simulink model "WAMVmodel_2017b"  (R2017b)
settings: Solver=ode23  StartTime=0.0  StopTime=param.tf  MaxStep=0.1  RelTol=1e-4  EnableMultiTasking=on
undefined symbols (not defined in the file or in its folder): param
settings Model: Creator=tristan  LastModifiedBy=masom
settings DataIOCC: LimitDataPoints=on  SaveFormat=Array  SignalLoggingSaveFormat=ModelDataLogs
settings OptimizationCC: ExpressionDepthLimit=2147483647  LifeSpan=inf
settings DebuggingCC: UnderspecifiedInitializationDetection=Classic  MergeDetectMultiDrivingBlocksExec=none  SolverPrmCheckMsg=warning  FcnCallInpInsideContextMsg=warning  StateNameClashWarn=warning  SFUnexpectedBacktrackingDiag=warning  SFNoUnconditionalDefaultTransitionDiag=warning  SFExecutionAtInitializationDiag=none
settings HardwareCC: ProdBitPerPointer=32  ProdBitPerSizeT=32  ProdBitPerPtrDiffT=32  ProdLargestAtomicFloat=None  ProdIntDivRoundTo=Undefined  ProdEndianess=Unspecified  ProdWordSize=32  ProdHWDeviceType=32-bit Generic
settings ModelReferenceCC: PropagateSignalLabelsOutOfModel=off
settings CodeAppCC: StateflowObjectComments=on
settings GRTTargetCC: TargetLangStandard=C89/C90 (ANSI)  GeneratePreprocessorConditionals=Disable all  CombineOutputUpdateFcns=off  GRTInterface=on
settings ConfigComp: CovMetricSettings=dw  CovHtmlReporting=on  CovSaveCumulativeToWorkspaceVar=on  CovSaveSingleToWorkspaceVar=on  CovExternalEMLEnable=off

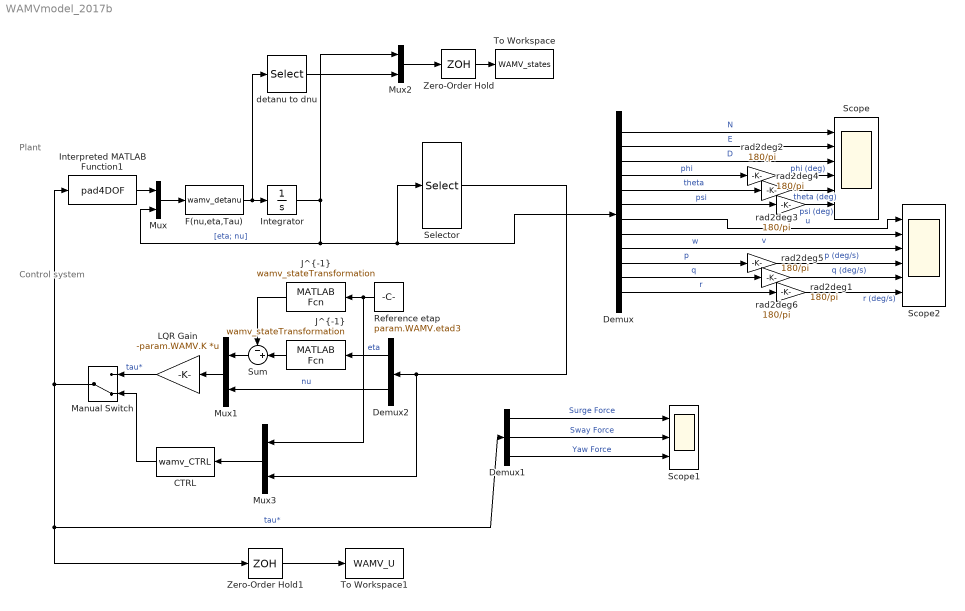
== system WAMVmodel_2017b ==
  note: Control system
  note: Plant
  CTRL : MATLABFcn  MATLABFcn=wamv_CTRL  OutputDimensions=3
  Demux : Demux  Outputs=12
  Demux1 : Demux  Outputs=3
  Demux2 : Demux  Outputs=[3,3]
  F(nu,eta,Tau) : MATLABFcn  MATLABFcn=wamv_detanu  OutputDimensions=12
  Integrator : Integrator  InitialCondition=param.WAMV.etai
  Interpreted MATLAB Function1 : MATLABFcn  MATLABFcn=pad4DOF  OutputDimensions=6
  "J^{-1}" : MATLABFcn  MATLABFcn=wamv_stateTransformation  OutputDimensions=3
  "J^{-1} " : MATLABFcn  MATLABFcn=wamv_stateTransformation  OutputDimensions=3
  LQR Gain : Gain  Gain=-param.WAMV.K  Multiplication=Matrix(K*u)
  Manual Switch : ManualSwitch  CurrentSetting=0
  Mux{,1..3} (4 alike) : Mux  Inputs=2
  Reference etap : Constant  Value=param.WAMV.etad3
  Scope : Scope  NumInputPorts=6
  Scope1 : Scope  NumInputPorts=3
  Scope2 : Scope  NumInputPorts=6
  Selector : Selector  InputPortWidth=12  IndexOptions=Index vector (dialog)  Indices=[1 2 6 7 8 12]  OutputSizes=1
  Sum : Sum  Inputs=-+|
  To Workspace : ToWorkspace  VariableName=WAMV_states  SaveFormat=Timeseries  SampleTime=-1
  To Workspace1 : ToWorkspace  VariableName=WAMV_U  SaveFormat=Timeseries  SampleTime=-1
  Zero-Order Hold : ZeroOrderHold  SampleTime=1/param.sensor_sample_rate
  Zero-Order Hold1 : ZeroOrderHold  SampleTime=1/param.sensor_sample_rate
  detanu to dnu : Selector  InputPortWidth=12  IndexOptions=Index vector (dialog)  Indices=[7:12]  OutputSizes=1
  rad2deg{1..6} (6 alike) : Gain  Gain=180/pi
  wires:
  Manual Switch/1 -> Interpreted MATLAB Function1/1, Demux1/1, Zero-Order Hold1/1  "tau*"
  Demux1/1 -> Scope1/1  "Surge Force"
  Demux1/2 -> Scope1/2  "Sway Force"
  Mux/1 -> F(nu,eta,Tau)/1
  F(nu,eta,Tau)/1 -> detanu to dnu/1, Integrator/1
  Integrator/1 -> Mux/2, Demux/1, Selector/1, Mux2/1  "[eta; nu]"
  Demux2/2 -> Mux1/2  "nu"
  Mux1/1 -> LQR Gain/1
  Demux1/3 -> Scope1/3  "Yaw Force"
  "J^{-1}"/1 -> Sum/2
  Reference etap/1 -> Mux3/1, "J^{-1} "/1
  Demux2/1 -> "J^{-1}"/1  "eta"
  Sum/1 -> Mux1/1
  "J^{-1} "/1 -> Sum/1
  Selector/1 -> Mux3/2, Demux2/1
  Demux/1 -> Scope/1  "N"
  Demux/2 -> Scope/2  "E"
  Demux/3 -> Scope/3  "D"
  Demux/4 -> rad2deg2/1  "phi"
  Demux/5 -> rad2deg3/1  "theta"
  Demux/6 -> rad2deg4/1  "psi"
  Demux/12 -> rad2deg1/1  "r"
  Demux/11 -> rad2deg6/1  "q"
  Demux/8 -> Scope2/2  "v"
  Demux/10 -> rad2deg5/1  "p"
  Demux/9 -> Scope2/3  "w"
  Demux/7 -> Scope2/1  "u"
  rad2deg2/1 -> Scope/4  "phi (deg)"
  rad2deg3/1 -> Scope/5  "theta (deg)"
  rad2deg4/1 -> Scope/6  "psi (deg)"
  rad2deg5/1 -> Scope2/4  "p (deg/s)"
  rad2deg6/1 -> Scope2/5  "q (deg/s)"
  rad2deg1/1 -> Scope2/6  "r (deg/s)"
  Interpreted MATLAB Function1/1 -> Mux/1
  Mux2/1 -> Zero-Order Hold/1
  Zero-Order Hold/1 -> To Workspace/1
  detanu to dnu/1 -> Mux2/2
  Zero-Order Hold1/1 -> To Workspace1/1
  LQR Gain/1 -> Manual Switch/1  "tau*"
  CTRL/1 -> Manual Switch/2
  Mux3/1 -> CTRL/1
